simulink model "disturbance_rejection"  (Simulink 8.7)
settings: Solver=ode45  StartTime=0.0  StopTime=2.0  RelTol=1e-3
settings Model: Creator=eechris  LastModifiedBy=eechris
settings DataIOCC: SignalLoggingSaveFormat=ModelDataLogs
settings OptimizationCC: ExpressionDepthLimit=2147483647
settings DebuggingCC: SolverPrmCheckMsg=warning  FcnCallInpInsideContextMsg=UseLocalSettings  StateNameClashWarn=warning
settings GRTTargetCC: CombineOutputUpdateFcns=off  GRTInterface=on

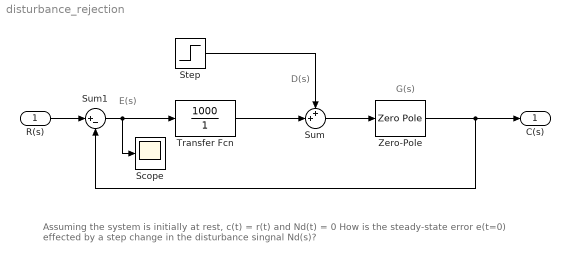
== system disturbance_rejection ==
  note: E(s)
  note: D(s)
  note: G(s)
  note: Assuming the system is initially at rest, c(t) = r(t) and Nd(t) = 0
      | How is the steady-state error e(t=0) effected by a step change in the disturbance singnal Nd(s)?
  R(s) : Inport
  Scope : Scope
  Step : Step  Time=0  SampleTime=0
  Sum : Sum  Inputs=++|
  Sum1 : Sum  Inputs=|+-
  Transfer Fcn : TransferFcn  Numerator=[1000]  Denominator=1
  Zero-Pole : ZeroPole  Zeros=[]  Poles=[0 -25]  Gain=1
  C(s) : Outport
  wires:
  Transfer Fcn/1 -> Sum/2
  R(s)/1 -> Sum1/1
  Sum1/1 -> Scope/1, Transfer Fcn/1
  Sum/1 -> Zero-Pole/1
  Zero-Pole/1 -> C(s)/1, Sum1/2
  Step/1 -> Sum/1
